simulink model "rtwdemo_filepart"  (Simulink 7.6)
settings: Solver=FixedStepDiscrete  StartTime=0.0  StopTime=10.0  RelTol=1e-3  SampleTimeConstraint=STIndependent
libraries: rtwdemowidgets x2
Description:
  | File Packaging for Atomic Subsystems (Code Only)
settings Model: Creator=The MathWorks Inc.  ExtModeAutoUpdateStatusClock=off
settings DataIOCC: SaveOutput=off  SaveTime=off  SignalLoggingName=sigsOut
settings OptimizationCC: InlineParams=on  InlineInvariantSignals=on  StateBitsets=on  DataBitsets=on  UseTempVars=on  EfficientFloat2IntCast=on  EfficientMapNaN2IntZero=off  BufferReusableBoundary=off
settings DebuggingCC: CheckExecutionContextPreStartOutputMsg=on  CheckExecutionContextRuntimeOutputMsg=on  SolverPrmCheckMsg=none  StrictBusMsg=ErrorOnBusTreatedAsVector
settings HardwareCC: ProdIntDivRoundTo=Zero  ProdEndianess=LittleEndian  ProdHWDeviceType=Generic->32-bit Embedded Processor  TargetHWDeviceType=Generic->32-bit Embedded Processor
settings RTWCC: TLCOptions=-p0 -aWarnNonSaturatedBlocks=0  GenerateReport=on  RTWVerbose=off  ProcessScript=grt_make_rtw_hook  LaunchReport=on
settings CodeAppCC: ForceParamTrailComments=on
settings GRTTargetCC: TargetFcnLib=ansi_tfl_tmw.mat

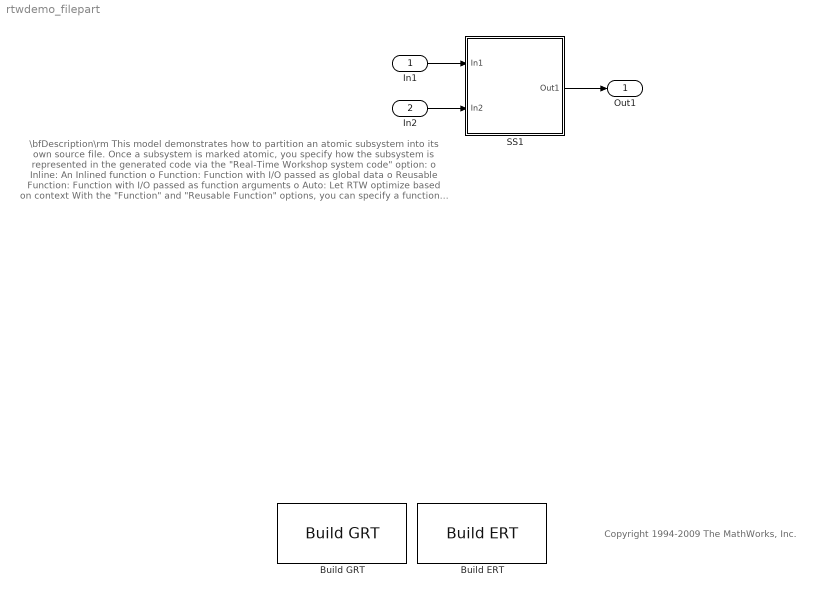
== system rtwdemo_filepart ==
  note: \bfDescription\rm
      | This model demonstrates how to partition an atomic subsystem into its own source file.  Once a
      | subsystem is marked atomic, you specify how the subsystem is represented in the generated code
      | via the "Real-Time Workshop system code" option:
      |
      | o  Inline: An Inlined function
      | o  Function: Function with I/O passed as global data
      | o  Reusable Function: Function with I/O passed as function arguments
      | o  Auto: Let RTW optimize based on context
      |
      | With the "Function" and "Reusable Function" options,  you can specify a function and file name via
      | "Real-Time Workshop function name" and "Real-Time Workshop file name," respectively.  Here,
      | SS1 is configured as "Reusable Function" with function name "myfun" and file name "myfile".
      |
      | \bfInstructions\rm
      | 1. To see the subsystem parameters, right-click the subsystem block and select "SubSystem Parameters."
      | 2. Generate code by double-clicking one of the blue buttons below.  An HTML report appears automatically.
      |
      | \bfNote\rm
      | This capability only partitions the code for a subsystem.  The data is declared and owned by
      | the parent model.  For full system encapsulation (i.e., data and functions), use Model Reference.
  note: Copyright 1994-2009 The MathWorks, Inc.
  In1 : Inport  OutDataTypeStr=double  PortDimensions=1
  In2 : Inport  Port=2  OutDataTypeStr=double  PortDimensions=1
  Build ERT : rtwdemowidgets/Build ERT  SystemSampleTime=-1  attrib_overrides={'ERTFilePackagingFormat'}
  Build GRT : rtwdemowidgets/Build GRT  SystemSampleTime=-1  attrib_overrides={}
  SS1 : Subsystem  TreatAsAtomicUnit=on  RTWFcnName=myfun  RTWFileName=myfile
      settings: RTWFcnNameOpts=User specified  RTWFileNameOpts=User specified
  Out1 : Outport
  wires:
  SS1/1(Out1) -> Out1/1
  In2/1 -> SS1/2(In2)
  In1/1 -> SS1/1(In1)

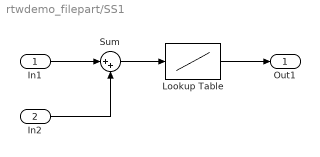
== system rtwdemo_filepart/SS1 ==
  In1 : Inport
  In2 : Inport  Port=2
  Lookup Table : Lookup  InputValues=[-5:5]  Table=tanh([-5:5])
  Sum : Sum  Inputs=|++
  Out1 : Outport
  wires:
  In1/1 -> Sum/1
  Lookup Table/1 -> Out1/1
  In2/1 -> Sum/2
  Sum/1 -> Lookup Table/1
